simulink library "MISC"  (R2019a)
settings: Solver=VariableStepAuto  StartTime=0.0  StopTime=10.0  RelTol=1e-3
libraries: xbsIndex_r4 x6
settings Model: Creator=mybur  LastModifiedBy=Ross Donnachie

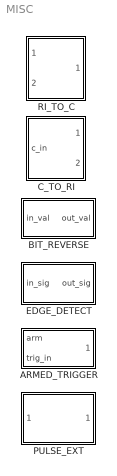
== system MISC ==
  ARMED_TRIGGER : Subsystem
      mask DialogControl DescTextVar Prompt: Makes a boolean trigger signal armable.
  BIT_REVERSE : Subsystem  mask{is_async=on}
      mask prompts: is_async "Asynchronous"
      mask init:
      | Simulink.Block.eval([gcb, '/bit_reverse']);
  C_TO_RI : Subsystem  mask{bit_width=4, bin_pt=0, is_async=off}
      mask prompts: bit_width "Bit Width"; bin_pt "Binary Point"; is_async "Asynchronous"
      mask init:
      | Simulink.Block.eval([gcb, '/c_to_ri']);
  EDGE_DETECT : Subsystem  mask{edge_type="rising", output_pol="high"}
      mask prompts: edge_type "Edge type to detect"; output_pol "Output polarity"
      mask init:
      | Simulink.Block.eval([gcb, '/edge_detect']);
      mask TypeOptions edge_type: "rising" | "falling" | "both"
      mask TypeOptions output_pol: "high" | "low"
      mask DialogControl DescTextVar Prompt: Detect input signal edges. Output is active for one-cycle after each edge of the specified type (i.e. rising, falling or both).
  PULSE_EXT : Subsystem  mask{extension=1}
      mask prompts: extension "How many clock cycles to extend the pulse-high by."
      mask DialogControl DescTextVar Prompt: Extends a boolean signal to be high for the specified number of clocks after the last high input.
  RI_TO_C : Subsystem  mask(ri_to_c){is_async=on}
      mask prompts: is_async "Asynchronous"
      mask help:
      | Concatenates real and imaginary inputs into a complex output.
      | Useful for simplifying interconnects.
      | See also: Complex to Real-Imag (c_to_ri).
      mask init:
      | Simulink.Block.eval([gcb, '/ri_to_c']);

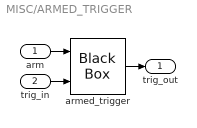
== system MISC/ARMED_TRIGGER ==
  arm : Inport
  trig_in : Inport  Port=2
  armed_trigger : xbsIndex_r4/Black Box  init_code=armed_trigger_config  sim_method=ISE Simulator  verbose=off  block_type=blackbox2
  trig_out : Outport
  wires:
  armed_trigger/1 -> trig_out/1
  trig_in/1 -> armed_trigger/2
  arm/1 -> armed_trigger/1

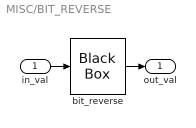
== system MISC/BIT_REVERSE ==
  in_val : Inport
  bit_reverse : xbsIndex_r4/Black Box  init_code=bit_reverse_config  sim_method=ISE Simulator  verbose=off  block_type=blackbox2
  out_val : Outport
  wires:
  in_val/1 -> bit_reverse/1
  bit_reverse/1 -> out_val/1

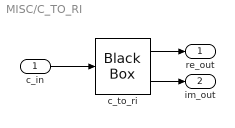
== system MISC/C_TO_RI ==
  c_in : Inport
  c_to_ri : xbsIndex_r4/Black Box  init_code=c_to_ri_config  sim_method=ISE Simulator  verbose=off  block_type=blackbox2
  re_out : Outport
  im_out : Outport  Port=2
  wires:
  c_to_ri/2 -> im_out/1
  c_to_ri/1 -> re_out/1
  c_in/1 -> c_to_ri/1

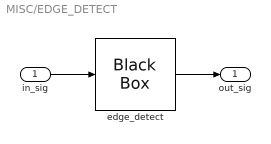
== system MISC/EDGE_DETECT ==
  in_sig : Inport
  edge_detect : xbsIndex_r4/Black Box  init_code=edge_detect_config  sim_method=ISE Simulator  verbose=off  block_type=blackbox2
  out_sig : Outport
  wires:
  in_sig/1 -> edge_detect/1
  edge_detect/1 -> out_sig/1

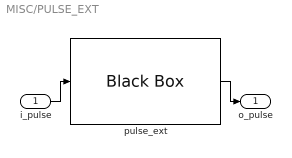
== system MISC/PULSE_EXT ==
  i_pulse : Inport
  pulse_ext : xbsIndex_r4/Black Box  init_code=pulse_ext_config  sim_method=ISE Simulator  verbose=off  block_type=blackbox2
  o_pulse : Outport
  wires:
  pulse_ext/1 -> o_pulse/1
  i_pulse/1 -> pulse_ext/1

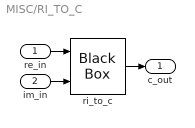
== system MISC/RI_TO_C ==
  re_in : Inport
  im_in : Inport  Port=2
  ri_to_c : xbsIndex_r4/Black Box  init_code=ri_to_c_config  sim_method=ISE Simulator  verbose=off  block_type=blackbox2
  c_out : Outport
  wires:
  im_in/1 -> ri_to_c/2
  re_in/1 -> ri_to_c/1
  ri_to_c/1 -> c_out/1
